simulink model "simulink_estanques"  (R2021a)
settings: Solver=ode1  StartTime=0.0  StopTime=5  FixedStep=0.001  RelTol=1e-3
settings Model: Creator=danie  LastModifiedBy=Agus

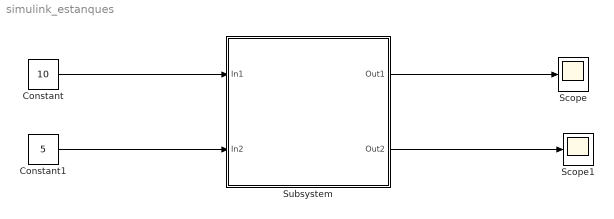
== system simulink_estanques ==
  Constant : Constant  Value=10
  Constant1 : Constant  Value=5
  Scope : Scope
  Scope1 : Scope
  Subsystem : Subsystem  mask{K=15, A=100, h10=14, h20=10}
      mask prompts: K "constante de no se qué"; A "Área"; h10 "altura10"; h20 "alturah20"
      mask Display:
      | port_label('input',1,'q1')
      | port_label('input',2,'q2')
      | port_label('output',1,'h1')
      | port_label('output',2,'h2')
      | fprintf('Sistema no lineal')
  wires:
  Constant/1 -> Subsystem/1(In1)
  Constant1/1 -> Subsystem/2(In2)
  Subsystem/1(Out1) -> Scope/1
  Subsystem/2(Out2) -> Scope1/1

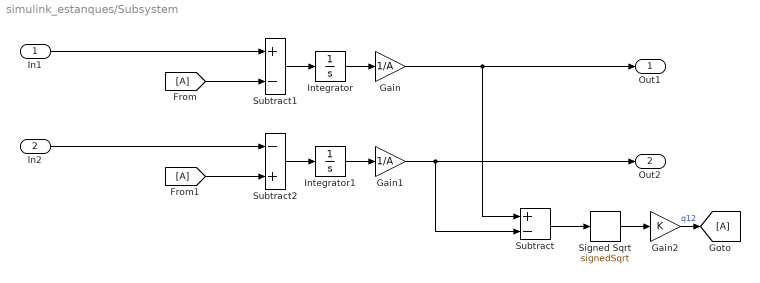
== system simulink_estanques/Subsystem ==
  In1 : Inport
  In2 : Inport  Port=2
  Gain : Gain  Gain=1/A
  Gain1 : Gain  Gain=1/A
  Gain2 : Gain  Gain=K
  Integrator : Integrator  InitialCondition=h10
  Integrator1 : Integrator  InitialCondition=h20
  Signed Sqrt : Sqrt  Operator=signedSqrt  SaturateOnIntegerOverflow=on
  Subtract : Sum  Inputs=+-
  Subtract1 : Sum  Inputs=+-
  Subtract2 : Sum  Inputs=-+
  Out1 : Outport
  Out2 : Outport  Port=2
  wires:
  Subtract/1 -> Signed Sqrt/1
  Signed Sqrt/1 -> Gain2/1
  In1/1 -> Subtract1/1
  Gain2/1 -> [A]  "q12"
  [A] -> Subtract1/2
  Subtract1/1 -> Integrator/1
  Integrator/1 -> Gain/1
  Gain/1 -> Subtract/1, Out1/1
  [A] -> Subtract2/2
  In2/1 -> Subtract2/1
  Subtract2/1 -> Integrator1/1
  Integrator1/1 -> Gain1/1
  Gain1/1 -> Subtract/2, Out2/1
